simulink model "SingleAGVSimpleModel"  (R2019b)
settings: Solver=VariableStepAuto  StartTime=0.0  StopTime=300  RelTol=1e-3
values from neighbouring files (symbols this model uses):
  n = Datesize(1,1)    [AGVPlot.m]
undefined symbols (not defined in the file or in its folder): m, sigbuilder_block
settings Model: PacingRate=2  Creator=Khaled  LastModifiedBy=Khaled

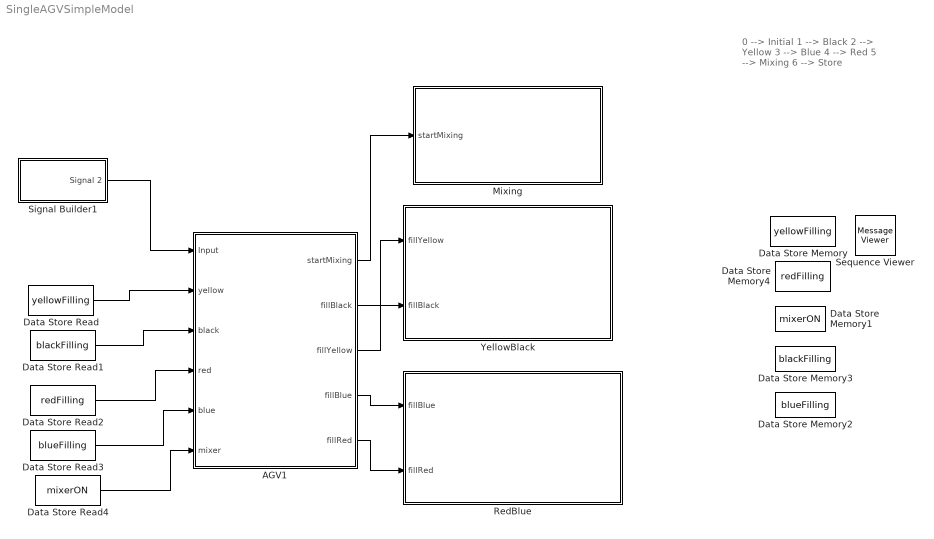
== system SingleAGVSimpleModel ==
  note: 0 --> Initial
      | 1 --> Black
      | 2 --> Yellow
      | 3 --> Blue
      | 4 --> Red
      | 5 --> Mixing
      | 6 --> Store
  AGV1 : Stateflow chart  BlockKeywords=__PRM__SERIALIZED__DATA__:Stateflow Chart,Stateflow Diagram  TreatAsAtomicUnit=on
  Data Store Read : DataStoreRead  DataStoreName=yellowFilling
  Data Store Read1 : DataStoreRead  DataStoreName=blackFilling
  Data Store Read2 : DataStoreRead  DataStoreName=redFilling
  Data Store Read3 : DataStoreRead  DataStoreName=blueFilling
  Data Store Read4 : DataStoreRead  DataStoreName=mixerON
  Data Store Memory : DataStoreMemory  DataStoreName=yellowFilling  ReadBeforeWriteMsg=warning  WriteAfterWriteMsg=warning  WriteAfterReadMsg=warning  ShowAdditionalParam=off  OutDataTypeStr=double
  Data Store Memory1 : DataStoreMemory  DataStoreName=mixerON  ReadBeforeWriteMsg=warning  WriteAfterWriteMsg=warning  WriteAfterReadMsg=warning  ShowAdditionalParam=off  OutDataTypeStr=double
  Data Store Memory2 : DataStoreMemory  DataStoreName=blueFilling  ReadBeforeWriteMsg=warning  WriteAfterWriteMsg=warning  WriteAfterReadMsg=warning  ShowAdditionalParam=off  OutDataTypeStr=double
  Data Store Memory3 : DataStoreMemory  DataStoreName=blackFilling  ReadBeforeWriteMsg=warning  WriteAfterWriteMsg=warning  WriteAfterReadMsg=warning  ShowAdditionalParam=off  OutDataTypeStr=double
  Data Store Memory4 : DataStoreMemory  DataStoreName=redFilling  ReadBeforeWriteMsg=warning  WriteAfterWriteMsg=warning  WriteAfterReadMsg=warning  ShowAdditionalParam=off  OutDataTypeStr=double
  Mixing : Stateflow chart  BlockKeywords=__PRM__SERIALIZED__DATA__:Stateflow Chart,Stateflow Diagram  TreatAsAtomicUnit=on
  RedBlue : Stateflow chart  BlockKeywords=__PRM__SERIALIZED__DATA__:Stateflow Chart,Stateflow Diagram  TreatAsAtomicUnit=on
  Sequence Viewer : MessageViewer  History=1000  SavedRootId=#
  Signal Builder1 : Subsystem  Tag=STV Subsys  LoadFcn=sigbuilder_block('load');  StartFcn=sigbuilder_block('start');  StopFcn=sigbuilder_block('stop');  ClipboardFcn=sigbuilder_block('clipboard');  mask(Sigbuilder block){tuvar=[0:10]}
      mask help: Simulink:masks:SigbuilderBlock_MD
      mask init:
      | if ~strcmp(get_param(bdroot(gcbh),'SimulationStatus'),'stopped') tuvar = sigbuilder_block('maskInit'); end
      settings: CopyFcn=sigbuilder_block('copy');  DeleteFcn=sigbuilder_block('delete');  ModelCloseFcn=sigbuilder_block('modelClose');  PreSaveFcn=sigbuilder_block('preSave');  PauseFcn=sigbuilder_block('pause');  ContinueFcn=sigbuilder_block('continue');  NameChangeFcn=sigbuilder_block('namechange');  OpenFcn=sigbuilder_block('open',[5.4 30 1141.2 522.6 ]);  CloseFcn=sigbuilder_block('close');
      mask Display: plot(0, 0, 100, 100,[2, 2, 32, 32, 2], [68, 8, 8, 68, 68],[32, 2], [38, 38], [32, 19, 2],[53, 60, 44], [32, 17, 17, 2],[16, 16, 31, 31]);txt = getActiveGroup(gcbh);text(2, 100, txt,'verticalAlignment', 'top');
  YellowBlack : Stateflow chart  BlockKeywords=__PRM__SERIALIZED__DATA__:Stateflow Chart,Stateflow Diagram  TreatAsAtomicUnit=on
  wires:
  AGV1/4(fillBlue) -> RedBlue/1(fillBlue)
  Data Store Read1/1 -> AGV1/3(black)
  Data Store Read3/1 -> AGV1/5(blue)
  Data Store Read2/1 -> AGV1/4(red)
  Data Store Read/1 -> AGV1/2(yellow)
  AGV1/2(fillBlack) -> YellowBlack/2(fillBlack)
  AGV1/3(fillYellow) -> YellowBlack/1(fillYellow)
  AGV1/5(fillRed) -> RedBlue/2(fillRed)
  Data Store Read4/1 -> AGV1/6(mixer)
  AGV1/1(startMixing) -> Mixing/1(startMixing)
  Signal Builder1/1(Signal 2) -> AGV1/1(Input)

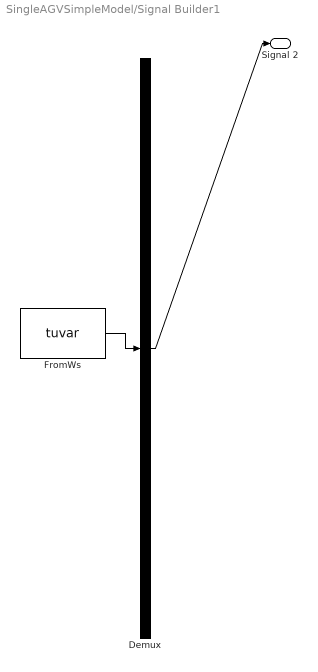
== system SingleAGVSimpleModel/Signal Builder1 ==
  Demux : Demux  Tag=STV Demux  Outputs=1
  FromWs : FromWorkspace  Tag=STV FromWs  VariableName=tuvar  SampleTime=0
      SigBuilderData=|
      | common.afterFinalStr = 'Extrapolate'
      | common.sampleTime = 0
      | dataSet.timeRange = [0 165]
      | dataSet.name = 'Group 1'
      | sbobj.Groups.Name = 'Group 1'
      | sbobj.Groups.Signals.Name = 'Signal 2'
      | sbobj.Groups.Signals.XData = [0 30 30 60 60 85 85 130.2 130.2 165]
      | sbobj.Groups.Signals.YData = [0 0 6 6 3 3 5 5 6 6]
      | sbobj.Groups.TimeRange = [0 165]
  Signal 2 : Outport  Tag=STV Outport
  wires:
  FromWs/1 -> Demux/1
  Demux/1 -> Signal 2/1

== stateflow chart SingleAGVSimpleModel/AGV1 ==
  state Black
    en:
    send(fillBlack);
  state Yellow
    en:
    send(fillYellow);
  state Storage
  state Transition
  state MixingStation
    en:
    send(startMixing);
  state InitPosition
  state Red
    en:
    send(fillRed);
  state Blue
    en:
    send(fillBlue);
  Yellow -> Black [order 1] : [Input==1]
  Black -> Yellow [order 1] : [Input==2]
  Transition -> Yellow [order 6] : [Input==2 && after(time,sec)]
  Black -> Transition [order 3] : [Input==5]...
      | /{time=T_YB_M}
  Transition -> Black [order 1] : [Input==1 && ...
      | after(time,sec)]
  Black -> Transition [order 2] : [Input==3 || Input==4]...
      | /{time=T_RB_YB}
  Yellow -> Transition [order 3] : [Input==5]...
      | /{time=T_YB_M}
  Yellow -> Transition [order 2] : [Input==3 || Input==4]...
      | /{time=T_RB_YB}
  Storage -> Transition [order 1] : [Input==1 || Input==2]/{time=T_S_YB}
  Storage -> Transition [order 2] : [Input==0]/{time=T_Init_S}
  Storage -> Transition [order 3] : [Input==3 || Input==4]/{time=T_S_RB}
  Transition -> Storage [order 3] : [Input==6 && after(time,sec)]
  Transition -> MixingStation [order 2] : [Input==5 && after(time,sec)]
  MixingStation -> Transition : [Input==6]/{time=T_M_S}
  InitPosition -> Transition : [Input==1 || Input==2 || Input==3 ||...
      |  Input==4|| Input==6]/{time=T_Init_S}
  Transition -> InitPosition [order 5] : [Input==0&&after(time,sec)]
  Transition -> Red [order 7] : [Input==4 &&...
      |  after(time,sec)]
  Red -> Transition [order 2] : [Input==5]...
      | /{time=T_RB_M}
  Red -> Transition [order 3] : [Input==2 || Input==1]...
      | /{time=T_RB_YB}
  Blue -> Transition [order 2] : [Input==1 || Input==2]...
      | /{time=T_RB_YB}
  Transition -> Blue [order 4] : [Input==3 && ...
      | after(time,sec)]
  Blue -> Transition [order 3] : [Input==5]...
      | /{time=T_RB_M}
  (default) -> InitPosition
  Blue -> Red [order 1] : [Input==4]
  Red -> Blue [order 1] : [Input==3]
  data: Input input; startMixing output boolean size=1; fillBlack output boolean size=1; fillYellow output boolean size=1; fillBlue output boolean size=1; fillRed output boolean size=1; yellow input; black input; red input; blue input; mixer input; T_YB_M constant double =10; T_RB_YB constant double =15; T_RB_M constant double =10; T_S_YB constant double =10; T_S_RB constant double =10; T_YB_RB constant double =15; T_M_S constant double =15; T_Init_S constant double =10; time local

== stateflow chart SingleAGVSimpleModel/Mixing ==
  state MixerOFF
    mixerON=0;
  state MixerON
    mixerON=1;
  MixerOFF -> MixerON : startMixing
  (default) -> MixerOFF
  MixerON -> MixerOFF : after(15,sec)
  data: startMixing input; mixerON data_store_memory

== stateflow chart SingleAGVSimpleModel/YellowBlack ==
  state Nofilling
    yellowFilling=0;
    blackFilling=0;
  state fillingBlack
    blackFilling=1;
  state FillingYellow
    yellowFilling=1;
  (default) -> Nofilling
  Nofilling -> fillingBlack [order 1] : fillBlack
  Nofilling -> FillingYellow [order 2] : fillYellow
  fillingBlack -> Nofilling : after(10,sec)
  FillingYellow -> Nofilling : after(10,sec)
  data: fillYellow input; fillBlack input; yellowFilling data_store_memory; blackFilling data_store_memory

== stateflow chart SingleAGVSimpleModel/RedBlue ==
  state Nofilling
    blueFilling=0;
    redFilling=0;
  state FillingRed
    redFilling=1;
  state FillingBlue
    blueFilling=1;
  (default) -> Nofilling
  Nofilling -> FillingRed [order 1] : fillRed
  Nofilling -> FillingBlue [order 2] : fillBlue
  FillingRed -> Nofilling : after(10,sec)
  FillingBlue -> Nofilling : after(10,sec)
  data: fillBlue input; fillRed input; blueFilling data_store_memory; redFilling data_store_memory
